simulink model "ControllerSuspActive"  (R2022b)
settings: Solver=ode14x  StartTime=0.0  StopTime=t(1,end)  FixedStep=t(1,end)-t(1,end-1)  RelTol=1e-3  EnableMultiTasking=on
values from neighbouring files (symbols this model uses):
  bs = 650    [MainCEoptCase3_FOPID.m]    (also in MainCEoptCase3_PID.m; MainGAoptCase3_FOPID.m; MainGAoptCase3_PID.m)
  Kd = x(3)    [MainCEoptCase3_FOPID.m]    (also in MainCEoptCase3_PID.m; MainGAoptCase3_FOPID.m; MainGAoptCase3_PID.m)
  Ki = x(2)    [MainCEoptCase3_FOPID.m]    (also in MainCEoptCase3_PID.m; MainGAoptCase3_FOPID.m; MainGAoptCase3_PID.m)
  Kp = x(1)    [MainCEoptCase3_FOPID.m]    (also in MainCEoptCase3_PID.m; MainGAoptCase3_FOPID.m; MainGAoptCase3_PID.m)
  ks = 10000    [MainCEoptCase3_FOPID.m]    (also in MainCEoptCase3_PID.m; MainGAoptCase3_FOPID.m; MainGAoptCase3_PID.m)
  ku = 200000    [MainCEoptCase3_FOPID.m]    (also in MainCEoptCase3_PID.m; MainGAoptCase3_FOPID.m; MainGAoptCase3_PID.m)
  ms = 250    [MainCEoptCase3_FOPID.m]    (also in MainCEoptCase3_PID.m; MainGAoptCase3_FOPID.m; MainGAoptCase3_PID.m)
  mu = 40    [MainCEoptCase3_FOPID.m]    (also in MainCEoptCase3_PID.m; MainGAoptCase3_FOPID.m; MainGAoptCase3_PID.m)
  r = 0    [MainCEoptCase3_FOPID.m]    (also in MainCEoptCase3_PID.m; MainGAoptCase3_FOPID.m; MainGAoptCase3_PID.m)
libraries: fod x2
settings Model: Creator=julio  LastModifiedBy=Ana Cláudia Rubim
settings SolverCC: AlgebraicLoopSolver=TrustRegion
settings DataIOCC: ReturnWorkspaceOutputs=off
settings OptimizationCC: LifeSpan=inf
settings DebuggingCC: UnconnectedInputMsg=warning  UnconnectedOutputMsg=warning  UnconnectedLineMsg=warning  SFUnexpectedBacktrackingDiag=warning  SFNoUnconditionalDefaultTransitionDiag=warning  SFMachineParentedDataDiag=warning  ArithmeticOperatorsInVariantConditions=warning
settings ModelReferenceCC: EnableRefExpFcnMdlSchedulingChecks=on
settings SFSimCC: SimUseLocalCustomCode=off  CustomCodeUndefinedFunction=UseInterfaceOnly
settings RTWCC: RTWUseLocalCustomCode=off
settings CodeAppCC: StateflowObjectComments=on
settings GRTTargetCC: TargetLangStandard=C89/C90 (ANSI)
settings ConfigComp: CovMetricSettings=dw  CovSaveCumulativeToWorkspaceVar=on  CovSaveSingleToWorkspaceVar=on  CovExternalEMLEnable=off

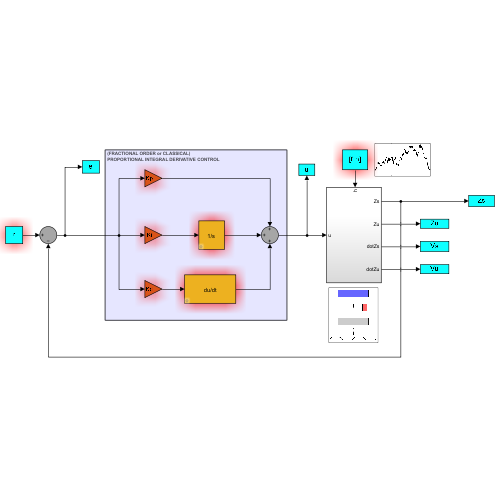
[thumbnail: Simulink's stored preview of the top-level diagram]
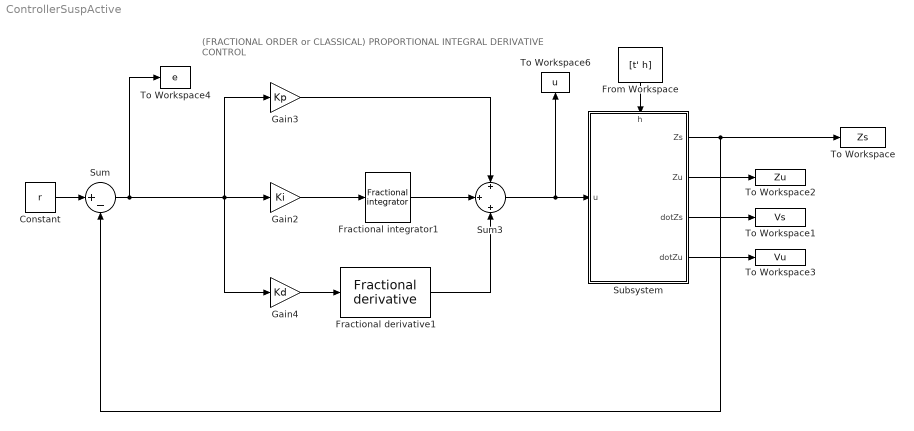
== system ControllerSuspActive ==
  note: (FRACTIONAL ORDER or CLASSICAL)
      | PROPORTIONAL INTEGRAL DERIVATIVE CONTROL
  Constant : Constant  Value=r
  Fractional derivative1 : fod/Fractional derivative  gam=OrderD  ww=[0.001; 1000]  n=5  nFod=off
      settings: SourceProductName=FOMCON Toolbox
  Fractional integrator1 : fod/Fractional integrator  gam=OrderI  ww=[0.001; 1000]  n=5  nFod=off
      settings: SourceProductName=FOMCON Toolbox
  From Workspace : FromWorkspace  VariableName=[t' h]
  Gain2 : Gain  Gain=Ki
  Gain3 : Gain  Gain=Kp
  Gain4 : Gain  Gain=Kd
  Subsystem : Subsystem
      settings: PortSchema="{\"entries\":[{\"content\":{\"sides\":[{\"content\":{\"connectorIds\":[\"In1\"]},\"type\":\"ConnectorPlacement.EquallySpacedRectSide\",\"uuid\":\"36165344-2bdb-4003-8a0b-4065714b97d9\"},{\"content\":{\"connectorIds\":[\"Out1\",\"Out2\",\"Out3\",\"Out4\"],\"side\":\"RIGHT\"},\"type\":\"ConnectorPlacement.EquallySpacedRectSide\",\"uuid\":\"3eb787ad-0d42-4ba9-bf4e-6a518a24b76f\"},{\"content\":{\"connectorIds\":[\"In2\"],\"side\":\"TOP\"},\"type\":\"ConnectorPlacement.EquallySpacedRectSide\",\"uuid\":\"d93f6027-d58d-4d70-b8be-8726d214fa0b\"}]},\"type\":\"ConnectorPlacement.EquallySpacedConnector\",\"uuid\":\"e8a050c0-c690-414a-b16b-6978cfe3ace7\"}],\"packageUris\":[\"http://schema.mathworks.com/mf0/Connector/R2020b\"],\"version\":\"1.0\"}"
  Sum : Sum  Inputs=|+-
  Sum3 : Sum  Inputs=+|+|+
  To Workspace : ToWorkspace  VariableName=Zs  SampleTime=-1
  To Workspace1 : ToWorkspace  VariableName=Vs  SampleTime=-1
  To Workspace2 : ToWorkspace  VariableName=Zu  SampleTime=-1
  To Workspace3 : ToWorkspace  VariableName=Vu  SampleTime=-1
  To Workspace4 : ToWorkspace  VariableName=e  SampleTime=-1
  To Workspace6 : ToWorkspace  VariableName=u  SampleTime=-1
  wires:
  Subsystem/1(Zs) -> To Workspace/1, Sum/2
  Constant/1 -> Sum/1
  Subsystem/2(Zu) -> To Workspace2/1
  Subsystem/3(dotZs) -> To Workspace1/1
  Subsystem/4(dotZu) -> To Workspace3/1
  Sum3/1 -> To Workspace6/1, Subsystem/1(u)
  Gain2/1 -> Fractional integrator1/1
  Gain3/1 -> Sum3/1
  Fractional integrator1/1 -> Sum3/2
  Gain4/1 -> Fractional derivative1/1
  Fractional derivative1/1 -> Sum3/3
  Sum/1 -> Gain3/1, Gain4/1, Gain2/1, To Workspace4/1
  From Workspace/1 -> Subsystem/2(h)

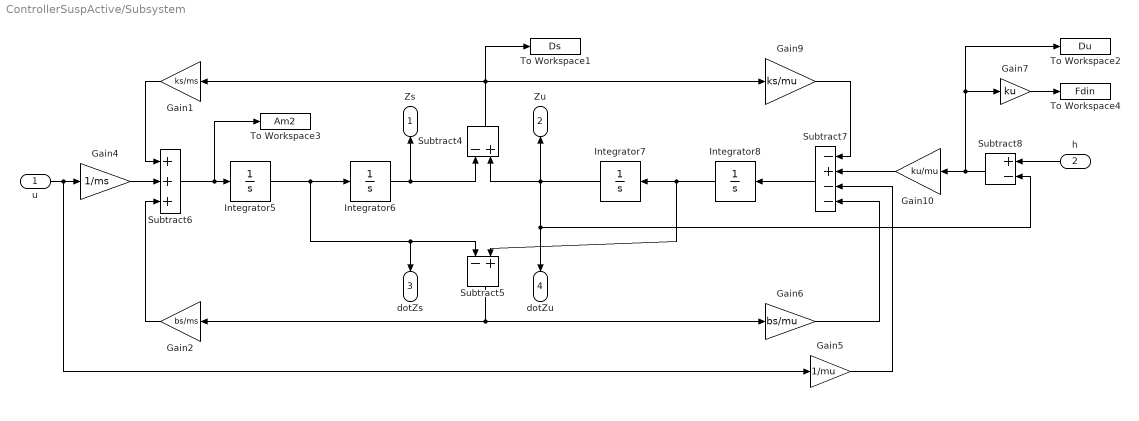
== system ControllerSuspActive/Subsystem ==
  u : Inport
  h : Inport  Port=2
  Gain1 : Gain  Gain=ks/ms
  Gain10 : Gain  Gain=ku/mu
  Gain2 : Gain  Gain=bs/ms
  Gain4 : Gain  Gain=1/ms
  Gain5 : Gain  Gain=1/mu
  Gain6 : Gain  Gain=bs/mu
  Gain7 : Gain  Gain=ku
  Gain9 : Gain  Gain=ks/mu
  Integrator{5..8} (4 alike) : Integrator
  Subtract4 : Sum  Inputs=-+
  Subtract5 : Sum  Inputs=-+
  Subtract6 : Sum  Inputs=+++
  Subtract7 : Sum  Inputs=-+--
  Subtract8 : Sum  Inputs=+-
  To Workspace1 : ToWorkspace  VariableName=Ds  SampleTime=-1
  To Workspace2 : ToWorkspace  VariableName=Du  SampleTime=-1
  To Workspace3 : ToWorkspace  VariableName=Am2  SampleTime=-1
  To Workspace4 : ToWorkspace  VariableName=Fdin  SampleTime=-1
  Zs : Outport
  Zu : Outport  Port=2
  dotZs : Outport  Port=3
  dotZu : Outport  Port=4
  wires:
  Integrator5/1 -> Subtract5/1, dotZs/1, Integrator6/1
  Integrator8/1 -> Subtract5/2, Integrator7/1
  Integrator7/1 -> Subtract8/2, dotZu/1, Subtract4/2, Zu/1
  Integrator6/1 -> Subtract4/1, Zs/1
  Subtract5/1 -> Gain6/1, Gain2/1
  Gain2/1 -> Subtract6/3
  Subtract6/1 -> To Workspace3/1, Integrator5/1
  Subtract7/1 -> Integrator8/1
  Gain9/1 -> Subtract7/1
  Gain6/1 -> Subtract7/4
  Gain10/1 -> Subtract7/2
  Gain1/1 -> Subtract6/1
  h/1 -> Subtract8/1
  Subtract4/1 -> To Workspace1/1, Gain9/1, Gain1/1
  Subtract8/1 -> Gain7/1, To Workspace2/1, Gain10/1
  u/1 -> Gain5/1, Gain4/1
  Gain4/1 -> Subtract6/2
  Gain5/1 -> Subtract7/3
  Gain7/1 -> To Workspace4/1
